simulink model "WoodandBerry1"  (Simulink 7.5)
settings: Solver=ode45  StartTime=0.0  StopTime=200  FixedStep=0.001  MaxStep=0.001  RelTol=1e-3
libraries: simulink_need_slupdate x2
settings Model: Creator=ARTURO  LastModifiedBy=ARTURO
settings OptimizationCC: ExpressionDepthLimit=128  InitFltsAndDblsToZero=on
settings DebuggingCC: SaveWithParameterizedLinksMsg=none  SignalResolutionControl=TryResolveAllWithWarning  MultiTaskDSMMsg=warning  MultiTaskCondExecSysMsg=none  StateNameClashWarn=none
settings CodeAppCC: CustomSymbolStrType=$N$R$M_T
settings GRTTargetCC: TargetFcnLib=ansi_tfl_tmw.mat  TargetFunctionLibrary=NOT IN USE  CPPClassGenCompliant=on

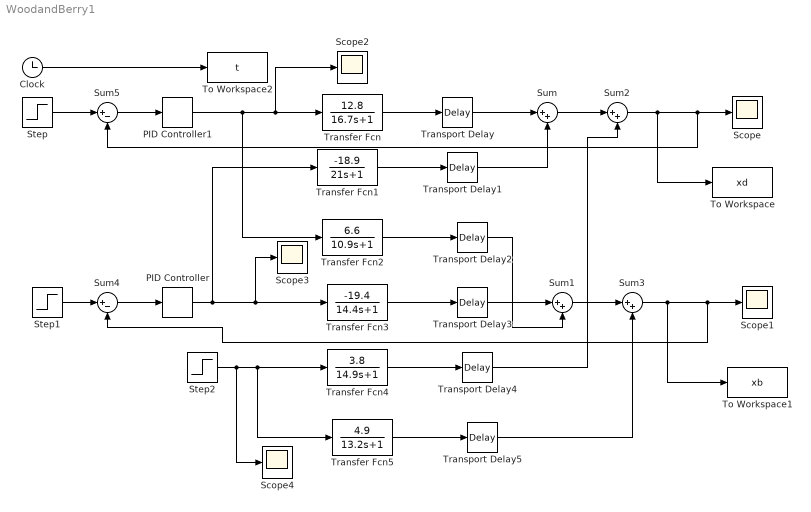
== system WoodandBerry1 ==
  Clock : Clock
      settings: Decimation=10
  PID Controller : simulink_need_slupdate/PID Controller  SystemSampleTime=-1  P=-0.075  I=-0.075/23.6  D=0
  PID Controller1 : simulink_need_slupdate/PID Controller  SystemSampleTime=-1  P=0.375  I=0.375/8.29  D=0
  Scope{,1..4} (5 alike) : Scope
      Scope settings: YMin=-0.004  YMax=-0.00025
      Scope1 settings: YMin=0.79  YMax=0.99
      Scope2 settings: YMin=-0.004  YMax=-0.00025  SaveName=Lsim  DataFormat=Array
      Scope3 settings: YMin=-0.004  YMax=-0.00025  SaveName=Vsim  DataFormat=Array
      Scope4 settings: YMin=-0.004  YMax=-0.00025  SaveName=Fsim  DataFormat=Array
  Step : Step  Time=0  After=0  SampleTime=0
  Step1 : Step  Time=0  SampleTime=0
  Step2 : Step  Time=20  After=0.05  SampleTime=0
  Sum{,1..3} (4 alike) : Sum  Inputs=|++
  Sum4 : Sum  Inputs=|+-
  Sum5 : Sum  Inputs=|+-
  To Workspace : ToWorkspace  VariableName=xd  SampleTime=-1  SaveFormat=Array
  To Workspace1 : ToWorkspace  VariableName=xb  SampleTime=-1  SaveFormat=Array
  To Workspace2 : ToWorkspace  VariableName=t  SampleTime=-1  SaveFormat=Array
  Transfer Fcn : TransferFcn  Numerator=12.8  Denominator=[16.7 1]
  Transfer Fcn1 : TransferFcn  Numerator=[-18.9]  Denominator=[21 1]
  Transfer Fcn2 : TransferFcn  Numerator=[6.6]  Denominator=[10.9 1]
  Transfer Fcn3 : TransferFcn  Numerator=-19.4  Denominator=[14.4 1]
  Transfer Fcn4 : TransferFcn  Numerator=3.8  Denominator=[14.9 1]
  Transfer Fcn5 : TransferFcn  Numerator=[4.9]  Denominator=[13.2 1]
  Transport Delay : TransportDelay  PadeOrder=5
  Transport Delay1 : TransportDelay  DelayTime=3  PadeOrder=5
  Transport Delay2 : TransportDelay  DelayTime=7  PadeOrder=5
  Transport Delay3 : TransportDelay  DelayTime=3  PadeOrder=5
  Transport Delay4 : TransportDelay  DelayTime=8  PadeOrder=5
  Transport Delay5 : TransportDelay  DelayTime=3  PadeOrder=5
  wires:
  Step2/1 -> Transfer Fcn4/1, Transfer Fcn5/1, Scope4/1
  PID Controller1/1 -> Scope2/1, Transfer Fcn/1, Transfer Fcn2/1
  PID Controller/1 -> Scope3/1, Transfer Fcn3/1, Transfer Fcn1/1
  Transfer Fcn/1 -> Transport Delay/1
  Transfer Fcn2/1 -> Transport Delay2/1
  Sum/1 -> Sum2/1
  Transfer Fcn1/1 -> Transport Delay1/1
  Transfer Fcn3/1 -> Transport Delay3/1
  Sum1/1 -> Sum3/1
  Transfer Fcn4/1 -> Transport Delay4/1
  Transfer Fcn5/1 -> Transport Delay5/1
  Sum4/1 -> PID Controller/1
  Sum5/1 -> PID Controller1/1
  Sum2/1 -> Sum5/2, Scope/1, To Workspace/1
  Sum3/1 -> Sum4/2, Scope1/1, To Workspace1/1
  Transport Delay/1 -> Sum/1
  Transport Delay3/1 -> Sum1/1
  Transport Delay4/1 -> Sum2/2
  Transport Delay5/1 -> Sum3/2
  Step/1 -> Sum5/1
  Step1/1 -> Sum4/1
  Transport Delay1/1 -> Sum/2
  Transport Delay2/1 -> Sum1/2
  Clock/1 -> To Workspace2/1
